simulink model "and_gate_model"  (R2023b)
settings: Solver=FixedStepAuto  StartTime=0.0  StopTime=10  FixedStep=1  RelTol=1e-3
settings Model: Creator=40662  LastModifiedBy=40476
settings OptimizationCC: DefaultParameterBehavior=Inlined  EnhancedBackFolding=on  PassReuseOutputArgsAs=Individual arguments  ZeroExternalMemoryAtStartup=off  ZeroInternalMemoryAtStartup=off  OptimizeBlockOrder=speed  DifferentSizesBufferReuse=on  OptimizationCustomize=off  EfficientTunableParamExpr=on
settings DebuggingCC: ParameterTunabilityLossMsg=error
settings SFSimCC: MATLABDynamicMemAlloc=off
settings RTWCC: Description=Embedded Coder  SystemTargetFile=ert.tlc  TemplateMakefile=ert_default_tmf
settings CodeAppCC: ForceParamTrailComments=on  IgnoreCustomStorageClasses=off  OperatorAnnotations=on  SimulinkDataObjDesc=on  SFDataObjDesc=on  InsertBlockDesc=on
settings ERTTargetCC: TargetLangStandard=C99 (ISO)  GenerateSampleERTMain=on  InlinedParameterPlacement=NonHierarchical  ERTCustomFileTemplate=example_file_process.tlc

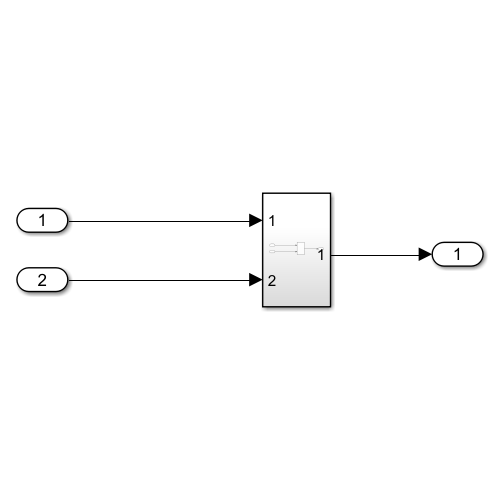
[thumbnail: Simulink's stored preview of the top-level diagram]
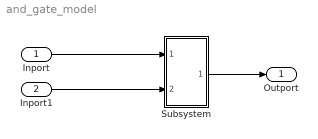
== system and_gate_model ==
  Inport : Inport  OutDataTypeStr=boolean
  Inport1 : Inport  Port=2  OutDataTypeStr=boolean
  Subsystem : Subsystem
  Outport : Outport  OutDataTypeStr=boolean
  wires:
  Inport/1 -> Subsystem/1(Inport)
  Inport1/1 -> Subsystem/2(Inport1)
  Subsystem/1(Outport) -> Outport/1

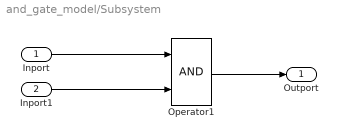
== system and_gate_model/Subsystem ==
  Inport : Inport  OutDataTypeStr=boolean
  Inport1 : Inport  Port=2  OutDataTypeStr=boolean
  Operator1 : Logic  AllPortsSameDT=off  OutDataTypeStr=boolean
  Outport : Outport  OutDataTypeStr=boolean
  wires:
  Operator1/1 -> Outport/1
  Inport/1 -> Operator1/1
  Inport1/1 -> Operator1/2
